simulink model "q3section3"  (R2020a)
settings: Solver=VariableStepAuto  StartTime=0.0  StopTime=10  RelTol=1e-3
values from neighbouring files (symbols this model uses):
  l = 280*10^(-6)    (= 0.00028)    [Q3B.m]
  N = 5    [Q3B.m]
libraries: cstblocks x2
settings Model: Creator=Nir Lalum  LastModifiedBy=Nir Lalum
settings SolverCC: ZeroCrossControl=EnableAll
settings SFSimCC: CustomCodeUndefinedFunction=UseInterfaceOnly

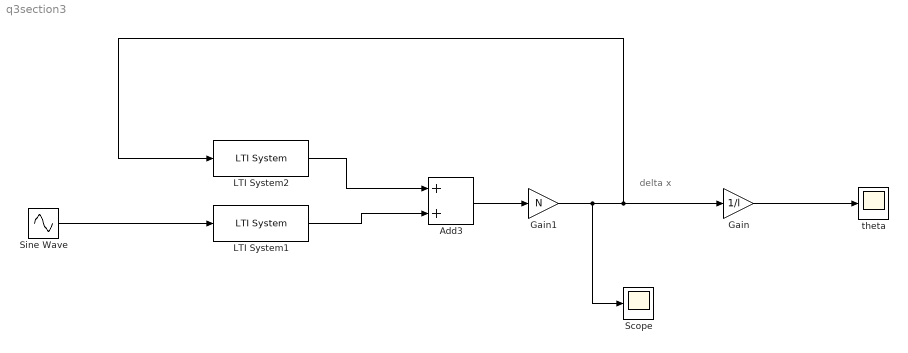
== system q3section3 ==
  note: delta x
  Add3 : Sum
  Gain : Gain  Gain=1/l
  Gain1 : Gain  Gain=N
  LTI System1 : cstblocks/LTI System  sys=Pv_x  IC=[]
  LTI System2 : cstblocks/LTI System  sys=Pf_tot  IC=[]
  Scope : Scope
  Sine Wave : Sin  Amplitude=491826381  Frequency=632  SampleTime=0
  theta : Scope
  wires:
  Add3/1 -> Gain1/1
  LTI System1/1 -> Add3/2
  Gain/1 -> theta/1
  LTI System2/1 -> Add3/1
  Sine Wave/1 -> LTI System1/1
  Gain1/1 -> LTI System2/1, Gain/1, Scope/1
